simulink model "test"  (R2017a)
settings: Solver=VariableStepAuto  StartTime=0.0  StopTime=10.0  RelTol=1e-3
undefined symbols (not defined in the file): Cwy1, Cwy2, Cx, Jyy, k1_k, k1_m, k2_k, k2_m, K_thruster, kc, L, lambda11, lambda55, m, T_thruster
libraries: simulink x5, powerlib_meascontrol x1
settings Model: Creator=Eugene  LastModifiedBy=Eugene

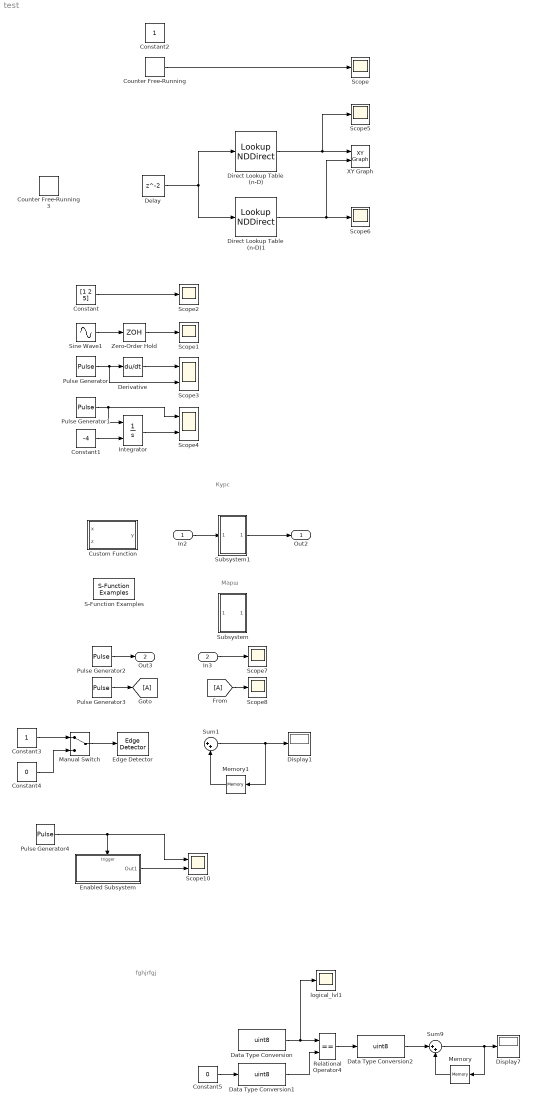
== system test ==
  note: fghjrfgj
  note: Курс
  note: Марш
  In2 : Inport
  In3 : Inport  Port=2
  Constant : Constant  Value=[1 2 5]
  Constant1 : Constant  Value=-4
  Constant2 : Constant
  Constant3 : Constant
  Constant4 : Constant  Value=0
  Constant5 : Constant  Value=0
  Counter Free-Running : simulink/Sources/Counter Free-Running  NumBits=16  tsamp=1
  Counter Free-Running3 : simulink/Sources/Counter Free-Running  NumBits=3  tsamp=1
  Custom Function : MATLAB Function  TreatAsAtomicUnit=on
  Data Type Conversion : DataTypeConversion  OutDataTypeStr=uint8
  Data Type Conversion1 : DataTypeConversion  OutDataTypeStr=uint8
  Data Type Conversion2 : DataTypeConversion  OutDataTypeStr=uint8
  Delay : Delay
  Derivative : Derivative
  Direct Lookup Table (n-D) : LookupNDDirect  NumberOfTableDimensions=1  Table=[0, 0, L, L, 2*L, 2*L, 3*L, 3*L]
  Direct Lookup Table (n-D)1 : LookupNDDirect  NumberOfTableDimensions=1  Table=[0, 25, 25, 0, 0, 25, 25, 0]
  Display1 : Display
  Display7 : Display
  Edge Detector : powerlib_meascontrol/Logic/Edge Detector  model=Falling  ic=0  Ts=0
      settings: SourceProductName=Simscape Power Systems  SourceProductBaseCode=PS
  Enabled Subsystem : Subsystem  TreatAsAtomicUnit=on
  Integrator : Integrator  InitialConditionSource=external
  Manual Switch : ManualSwitch
  Memory : Memory
  Memory1 : Memory
  Pulse Generator : DiscretePulseGenerator  PulseType=Time based  PulseWidth=5
  Pulse Generator{1..4} (4 alike) : DiscretePulseGenerator  PulseType=Time based  PulseWidth=50
  Relational Operator4 : RelationalOperator  Operator===  OutDataTypeStr=boolean  RndMeth=Simplest
  S-Function Examples : simulink/User-Defined Functions/S-Function Examples
      settings: SourceProductName=Simulink  SourceProductBaseCode=SL
  Scope{,1..2,5..8} (7 alike) : Scope
  Scope10 : Scope  NumInputPorts=2
  Scope3 : Scope  NumInputPorts=2
  Scope4 : Scope  NumInputPorts=2
  Sine Wave1 : Sin  SampleTime=0
  Subsystem : Subsystem
  Subsystem1 : Subsystem
  Sum1 : Sum  Inputs=|++
  Sum9 : Sum  Inputs=|++
  XY Graph : simulink/Sinks/XY Graph  xmin=-1  xmax=1  ymin=-1  ymax=1  st=-1
  Zero-Order Hold : ZeroOrderHold  SampleTime=-1
  logical_lvl1 : Scope
  Out2 : Outport
  Out3 : Outport  Port=2  SignalName=asd
  wires:
  Sine Wave1/1 -> Zero-Order Hold/1
  Zero-Order Hold/1 -> Scope1/1
  Constant/1 -> Scope2/1
  Derivative/1 -> Scope3/1
  Pulse Generator/1 -> Scope3/2, Derivative/1
  Pulse Generator1/1 -> Integrator/1, Scope4/1
  Constant1/1 -> Integrator/2
  Integrator/1 -> Scope4/2
  ? -> Delay/1
  Direct Lookup Table (n-D)1/1 -> XY Graph/2, Scope6/1
  Direct Lookup Table (n-D)/1 -> Scope5/1, XY Graph/1
  Delay/1 -> Direct Lookup Table (n-D)/1, Direct Lookup Table (n-D)1/1
  Counter Free-Running/1 -> Scope/1
  Subsystem1/1(Out2) -> Out2/1
  In2/1 -> Subsystem1/1(In2)
  Pulse Generator2/1 -> Out3/1
  In3/1 -> Scope7/1
  Pulse Generator3/1 -> [A]
  [A] -> Scope8/1
  Manual Switch/1 -> Edge Detector/1
  Constant3/1 -> Manual Switch/1
  Constant4/1 -> Manual Switch/2
  Memory1/1 -> Sum1/2
  Sum1/1 -> Display1/1, Memory1/1
  Enabled Subsystem/1(Out1) -> Scope10/2
  Pulse Generator4/1 -> Enabled Subsystem/Trigger, Scope10/1
  Constant5/1 -> Data Type Conversion1/1
  Data Type Conversion2/1 -> Sum9/1
  Data Type Conversion1/1 -> Relational Operator4/2
  Relational Operator4/1 -> Data Type Conversion2/1
  Data Type Conversion/1 -> logical_lvl1/1, Relational Operator4/1
  Memory/1 -> Sum9/2
  Sum9/1 -> Display7/1, Memory/1
  ? -> Data Type Conversion/1

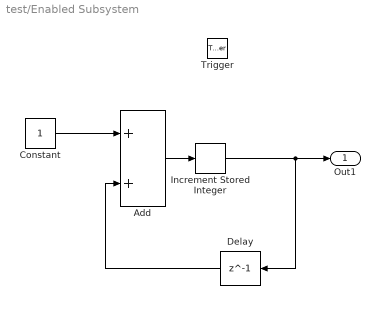
== system test/Enabled Subsystem ==
  Trigger : TriggerPort  TriggerType=falling  VariantControl=Variant  PortDimensions=1
  Add : Sum
  Constant : Constant
  Delay : Delay  DelayLength=1  InitialCondition=0
  Increment Stored Integer : simulink/Additional Math & Discrete/Additional Math: Increment - Decrement/Increment Stored Integer
      settings: SourceProductName=Simulink
  Out1 : Outport
  wires:
  Constant/1 -> Add/1
  Delay/1 -> Add/2
  Add/1 -> Increment Stored Integer/1
  Increment Stored Integer/1 -> Delay/1, Out1/1

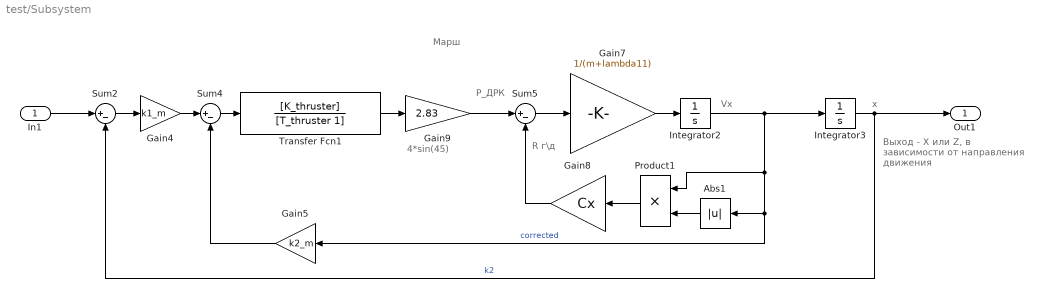
== system test/Subsystem ==
  note: Выход - X или Z, в зависимости от направления движения
  note: 4*sin(45)
  note: R г\д
  note: x
  note: Vx
  note: P_ДРК
  note: Марш
  In1 : Inport
  Abs1 : Abs
  Gain4 : Gain  Gain=k1_m
  Gain5 : Gain  Gain=k2_m
  Gain7 : Gain  Gain=1/(m+lambda11)
  Gain8 : Gain  Gain=Cx
  Gain9 : Gain  Gain=2.83
  Integrator2 : Integrator
  Integrator3 : Integrator
  Product1 : Product
  Sum2 : Sum  Inputs=|+-
  Sum4 : Sum  Inputs=|+-
  Sum5 : Sum  Inputs=|+-
  Transfer Fcn1 : TransferFcn  Numerator=[K_thruster]  Denominator=[T_thruster 1]
  Out1 : Outport
  wires:
  In1/1 -> Sum2/1
  Sum2/1 -> Gain4/1
  Product1/1 -> Gain8/1
  Gain7/1 -> Integrator2/1
  Gain8/1 -> Sum5/2
  Integrator2/1 -> Integrator3/1, Gain5/1, Abs1/1, Product1/1  "corrected"
  Transfer Fcn1/1 -> Gain9/1
  Gain4/1 -> Sum4/1
  Sum4/1 -> Transfer Fcn1/1
  Integrator3/1 -> Out1/1, Sum2/2  "k2"
  Sum5/1 -> Gain7/1
  Gain9/1 -> Sum5/1
  Gain5/1 -> Sum4/2
  Abs1/1 -> Product1/2

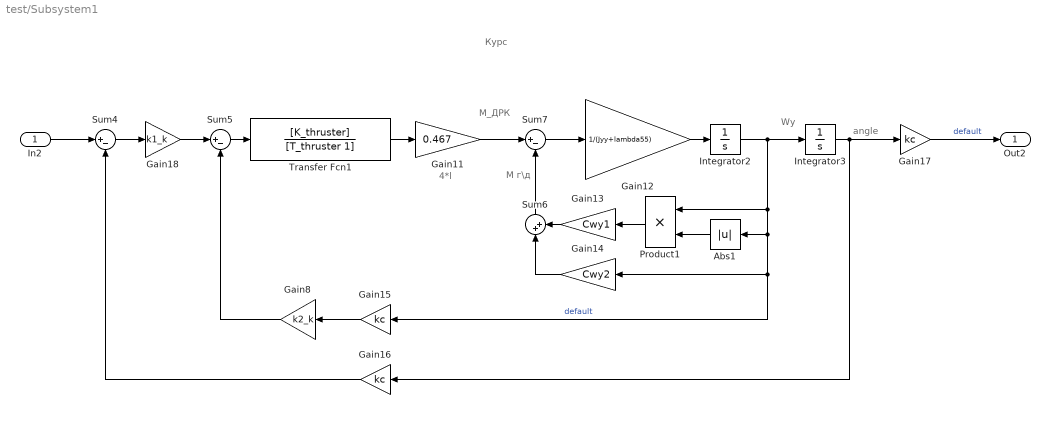
== system test/Subsystem1 ==
  note: M г\д
  note: M_ДРК
  note: angle
  note: Wy
  note: 4*l
  note: Курс
  In2 : Inport
  Abs1 : Abs
  Gain11 : Gain  Gain=0.467
  Gain12 : Gain  Gain=1/(Jyy+lambda55)
  Gain13 : Gain  Gain=Cwy1
  Gain14 : Gain  Gain=Cwy2
  Gain15 : Gain  Gain=kc
  Gain16 : Gain  Gain=kc
  Gain17 : Gain  Gain=kc
  Gain18 : Gain  Gain=k1_k
  Gain8 : Gain  Gain=k2_k
  Integrator2 : Integrator
  Integrator3 : Integrator
  Product1 : Product
  Sum4 : Sum  Inputs=|+-
  Sum5 : Sum  Inputs=|+-
  Sum6 : Sum  Inputs=|++
  Sum7 : Sum  Inputs=|+-
  Transfer Fcn1 : TransferFcn  Numerator=[K_thruster]  Denominator=[T_thruster 1]
  Out2 : Outport
  wires:
  Integrator3/1 -> Gain17/1, Gain16/1
  Product1/1 -> Gain13/1
  Integrator2/1 -> Integrator3/1, Product1/1, Abs1/1, Gain14/1, Gain15/1  "default"
  Gain15/1 -> Gain8/1
  Gain18/1 -> Sum5/1
  Sum7/1 -> Gain12/1
  Gain16/1 -> Sum4/2
  Sum5/1 -> Transfer Fcn1/1
  Gain12/1 -> Integrator2/1
  Abs1/1 -> Product1/2
  Gain14/1 -> Sum6/1
  Sum4/1 -> Gain18/1
  Gain11/1 -> Sum7/1
  Gain13/1 -> Sum6/2
  Transfer Fcn1/1 -> Gain11/1
  Sum6/1 -> Sum7/2
  Gain8/1 -> Sum5/2
  Gain17/1 -> Out2/1  "default"
  In2/1 -> Sum4/1

== matlab function test/Custom Function ==
  data: x input; y output; z input
function y = fcn(x, z)

y = x+z;
